simulink model "find_id_index_test"  (R2021b)
settings: Solver=VariableStepAuto  StartTime=0.0  StopTime=stop_time  RelTol=1e-3
libraries: dspsrcs4 x3
settings Model: Creator=torha  LastModifiedBy=torha
settings SolverCC: AlgebraicLoopSolver=TrustRegion
settings DebuggingCC: SFMachineParentedDataDiag=warning

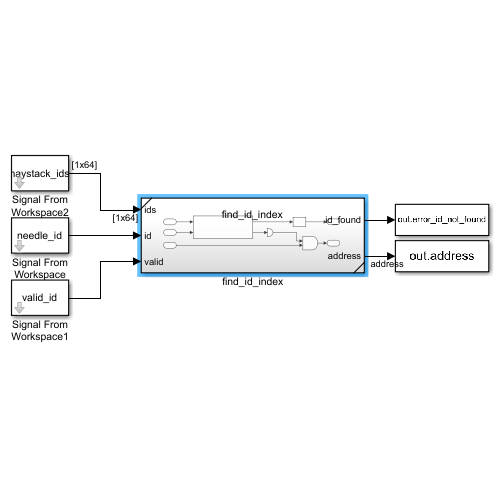
[thumbnail: Simulink's stored preview of the top-level diagram]
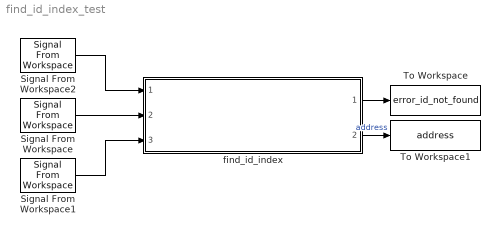
== system find_id_index_test ==
  Signal From Workspace : dspsrcs4/Signal From Workspace  X=needle_id  Ts=1  nsamps=1  OutputAfterFinalValue=Setting to zero  ignoreOrWarnInputAndFrameLengths=off  OutputFrames=off
  Signal From Workspace1 : dspsrcs4/Signal From Workspace  X=valid_id  Ts=1  nsamps=1  OutputAfterFinalValue=Setting to zero  ignoreOrWarnInputAndFrameLengths=off  OutputFrames=off
  Signal From Workspace2 : dspsrcs4/Signal From Workspace  X=haystack_ids  Ts=1  nsamps=1  OutputAfterFinalValue=Setting to zero  ignoreOrWarnInputAndFrameLengths=off  OutputFrames=off
  To Workspace : ToWorkspace  VariableName=error_id_not_found  SampleTime=-1
      settings: Save2DSignal=2-D array (concatenate along first dimension)
  To Workspace1 : ToWorkspace  VariableName=address  SampleTime=-1
      settings: Save2DSignal=2-D array (concatenate along first dimension)
  find_id_index : Subsystem  ReferencedSubsystem=find_id_index
  wires:
  Signal From Workspace/1 -> find_id_index/2
  Signal From Workspace1/1 -> find_id_index/3
  Signal From Workspace2/1 -> find_id_index/1
  find_id_index/1 -> To Workspace/1
  find_id_index/2 -> To Workspace1/1  "address"
